simulink model "sim"  (R2021a)
settings: Solver=VariableStepAuto  StartTime=0.0  StopTime=5  RelTol=1e-3
values from neighbouring files (symbols this model uses):
  A = [0,1,0,0;0,0,-9.41492892836899,0;0,0,0,1;0,0,-192.249289283690,0]    [sim_lqg.m]
  B = [0;141.136429339344;0;1411.36429339344]    [sim_lqg.m]
  C = [1,0,0,0]    [sim_lqg.m]
  Mean_v = mean(v)    [sim_lqg.m]
  Mean_w = mean(w)    [sim_lqg.m]
  Nbar = -inv(C*inv(A-B*K)*B)    [sim_lqg.m]
  Var_v = (std(v))^2    [sim_lqg.m]
  Var_w = (std(w))^2    [sim_lqg.m]
undefined symbols (not defined in the file or in its folder): K, L
settings Model: Creator=USUARIO  LastModifiedBy=USUARIO

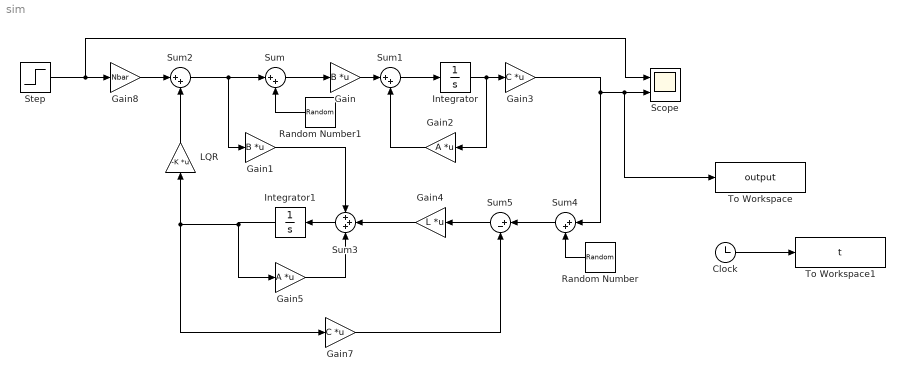
== system sim ==
  Clock : Clock
  Gain : Gain  Gain=B  Multiplication=Matrix(K*u)
  Gain1 : Gain  Gain=B  Multiplication=Matrix(K*u)
  Gain2 : Gain  Gain=A  Multiplication=Matrix(K*u)
  Gain3 : Gain  Gain=C  Multiplication=Matrix(K*u)
  Gain4 : Gain  Gain=L  Multiplication=Matrix(K*u)
  Gain5 : Gain  Gain=A  Multiplication=Matrix(K*u)
  Gain7 : Gain  Gain=C  Multiplication=Matrix(K*u)
  Gain8 : Gain  Gain=Nbar
  Integrator : Integrator
  Integrator1 : Integrator
  LQR : Gain  Gain=-K  Multiplication=Matrix(K*u)
  Random Number : RandomNumber  Mean=Mean_v  Variance=Var_v  SampleTime=0.1
  Random Number1 : RandomNumber  Mean=Mean_w  Variance=Var_w  SampleTime=0.1
  Scope : Scope  NumInputPorts=2
  Step : Step  SampleTime=0
  Sum{,1..2,4} (4 alike) : Sum  Inputs=|++
  Sum3 : Sum  Inputs=+++
  Sum5 : Sum  Inputs=|+-
  To Workspace : ToWorkspace  VariableName=output
  To Workspace1 : ToWorkspace  VariableName=t
  wires:
  Gain8/1 -> Sum2/1
  Gain2/1 -> Sum1/2
  Step/1 -> Gain8/1, Scope/1
  LQR/1 -> Sum2/2
  Gain4/1 -> Sum3/2
  Random Number/1 -> Sum4/2
  Gain5/1 -> Sum3/3
  Sum1/1 -> Integrator/1
  Sum5/1 -> Gain4/1
  Sum4/1 -> Sum5/1
  Random Number1/1 -> Sum/2
  Integrator/1 -> Gain3/1, Gain2/1
  Gain/1 -> Sum1/1
  Gain3/1 -> Sum4/1, To Workspace/1, Scope/2
  Integrator1/1 -> LQR/1, Gain7/1, Gain5/1
  Sum2/1 -> Gain1/1, Sum/1
  Sum3/1 -> Integrator1/1
  Sum/1 -> Gain/1
  Gain1/1 -> Sum3/1
  Gain7/1 -> Sum5/2
  Clock/1 -> To Workspace1/1
